simulink model "neurona"  (Simulink 7.5)
settings: Solver=ode45  StartTime=0.0  StopTime=2  RelTol=1e-3
undefined symbols (not defined in the file or in its folder): sigbuilder_block
settings Model: Creator=My Laptop  LastModifiedBy=My Laptop

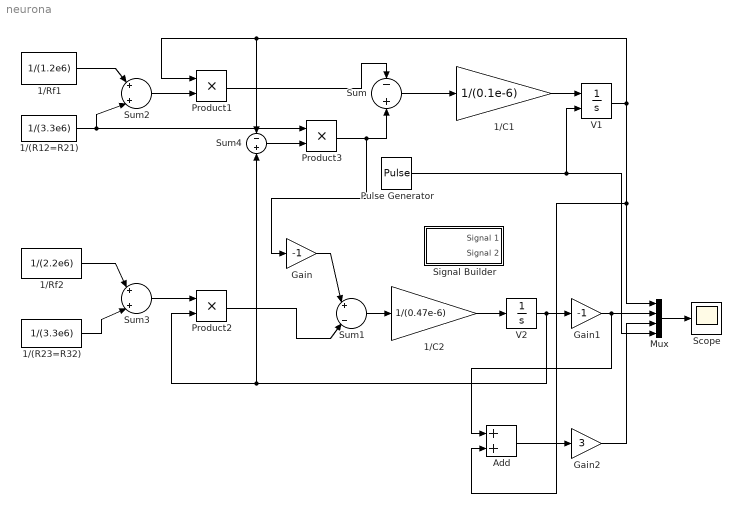
== system neurona ==
  1/(R12=R21) : Constant  Value=1/(3.3e6)  OutDataType=fixdt(1, 16)  OutScaling=2^0
  1/(R23=R32) : Constant  Value=1/(3.3e6)  OutDataType=fixdt(1, 16)  OutScaling=2^0
  1/C1 : Gain  Gain=1/(0.1e-6)  ParameterDataType=fixdt(1, 16)  ParameterScaling=2^0  OutDataType=fixdt(1, 16)  OutScaling=2^0
  1/C2 : Gain  Gain=1/(0.47e-6)  ParameterDataType=fixdt(1, 16)  ParameterScaling=2^0  OutDataType=fixdt(1, 16)  OutScaling=2^0
  1/Rf1 : Constant  Value=1/(1.2e6)  OutDataType=fixdt(1, 16)  OutScaling=2^0
  1/Rf2 : Constant  Value=1/(2.2e6)  OutDataType=fixdt(1, 16)  OutScaling=2^0
  Add : Sum  OutDataType=fixdt(1, 16)  OutScaling=2^-10
  Gain : Gain  Gain=-1  ParameterDataType=fixdt(1, 16)  ParameterScaling=2^0  OutDataType=fixdt(1, 16)  OutScaling=2^0
  Gain1 : Gain  Gain=-1  ParameterDataType=fixdt(1, 16)  ParameterScaling=2^0  OutDataType=fixdt(1, 16)  OutScaling=2^0
  Gain2 : Gain  Gain=3  ParameterDataType=fixdt(1, 16)  ParameterScaling=2^0  OutDataType=fixdt(1, 16)  OutScaling=2^0
  Mux : Mux
  Product1 : Product  OutDataType=fixdt(1, 16)  OutScaling=2^0  RndMeth=Zero
  Product2 : Product  OutDataType=fixdt(1, 16)  OutScaling=2^0  RndMeth=Zero
  Product3 : Product  OutDataType=fixdt(1, 16)  OutScaling=2^0  RndMeth=Zero
  Pulse Generator : DiscretePulseGenerator  PulseType=Time based  Amplitude=1  Period=1  PulseWidth=.1  PhaseDelay=0  SampleTime=1
  Scope : Scope
      settings: TimeRange=2  YMin=-1  YMax=1
  Signal Builder : Subsystem  Tag=STV Subsys  LoadFcn=sigbuilder_block('load');  StartFcn=sigbuilder_block('start');  StopFcn=sigbuilder_block('stop');  ClipboardFcn=sigbuilder_block('clipboard');  mask(Sigbuilder block){}
      mask help: Create and generate interchangeable groups of signals whose waveforms are piecewise linear.
      mask init:
      | if ~strcmp(get_param(bdroot(gcbh),'SimulationStatus'),'stopped') tuvar = sigbuilder_block('maskInit'); end
      settings: CopyFcn=sigbuilder_block('copy');  DeleteFcn=sigbuilder_block('delete');  ModelCloseFcn=sigbuilder_block('modelClose');  PreSaveFcn=sigbuilder_block('preSave');  NameChangeFcn=sigbuilder_block('namechange');  OpenFcn=sigbuilder_block('open',[437.25 120 550.5 394.5 ]);  CloseFcn=sigbuilder_block('close');
      mask Display: plot(0,0,100,100,[10,10,40,40,10],[80,20,20,80,80],[40,10],[50,50], [40,27,10],[65,72,56],[40,25,25,10],[28,28,43,43]);
  Sum : Sum  Inputs=-|+  OutDataType=fixdt(1, 16)  OutScaling=2^0
  Sum1 : Sum  Inputs=|+|-|  OutDataType=fixdt(1, 16)  OutScaling=2^0
  Sum2 : Sum  Inputs=|+|+|  OutDataType=fixdt(1, 16)  OutScaling=2^0
  Sum3 : Sum  Inputs=|+|+|  OutDataType=fixdt(1, 16)  OutScaling=2^0
  Sum4 : Sum  Inputs=-|+  OutDataType=fixdt(1, 16)  OutScaling=2^0
  V1 : Integrator  ExternalReset=level  InitialCondition=1
  V2 : Integrator
  wires:
  1/C1/1 -> V1/1
  Mux/1 -> Scope/1
  V1/1 -> Product1/1, Sum4/1, Add/2, Mux/1
  1/C2/1 -> V2/1
  Sum/1 -> 1/C1/1
  Sum1/1 -> 1/C2/1
  1/Rf1/1 -> Sum2/1
  1/(R12=R21)/1 -> Sum2/2, Product3/1
  1/Rf2/1 -> Sum3/1
  1/(R23=R32)/1 -> Sum3/2
  Sum2/1 -> Product1/2
  Sum3/1 -> Product2/1
  Product1/1 -> Sum/1
  Product2/1 -> Sum1/2
  Product3/1 -> Sum/2, Gain/1
  Gain/1 -> Sum1/1
  Sum4/1 -> Product3/2
  V2/1 -> Gain1/1, Product2/2, Sum4/2
  Gain1/1 -> Mux/2, Add/1
  Add/1 -> Gain2/1
  Gain2/1 -> Mux/3
  Pulse Generator/1 -> V1/2, Mux/4

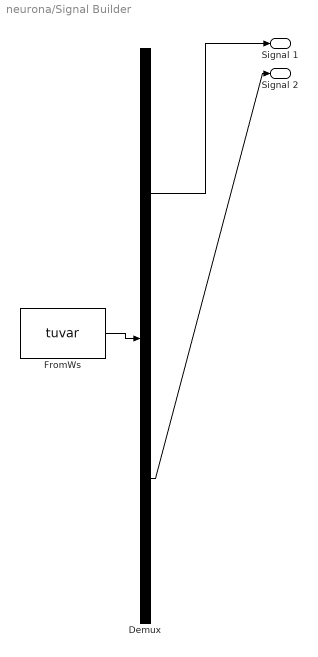
== system neurona/Signal Builder ==
  Demux : Demux  Tag=STV Demux  Outputs=2
  FromWs : FromWorkspace  Tag=STV FromWs  VariableName=tuvar  SampleTime=0  SigBuilderData=DataTag0  VnvData=DataTag1
      SigBuilderData=|
      | common.afterFinalStr = 'Extrapolate'
      | common.sampleTime = 0
      | dataSet.timeRange = [0 2]
      | dataSet.name = 'Group 1'
      | sbobj.Groups.Name = 'Group 1'
      | sbobj.Groups.Signals(1).Name = 'Signal 1'
      | sbobj.Groups.Signals(1).XData = [0 0.8 1 1.8 2]
      | sbobj.Groups.Signals(1).YData = [0 1 0 1 0]
      | sbobj.Groups.Signals(2).Name = 'Signal 2'
      | sbobj.Groups.Signals(2).XData = [0 1 1 2]
      | sbobj.Groups.Signals(2).YData = [0 2 0 2]
  Signal 1 : Outport  Tag=STV Outport  OutDataType=fixdt(1, 16)  OutScaling=2^0
  Signal 2 : Outport  Tag=STV Outport  Port=2
  wires:
  Demux/1 -> Signal 1/1
  FromWs/1 -> Demux/1
  Demux/2 -> Signal 2/1
